simulink model "simulink_pa_lqr_based"  (R2016b)
settings: Solver=FixedStepAuto  StartTime=0.0  StopTime=1  FixedStep=Splant  RelTol=1e-3
undefined symbols (not defined in the file): Ad_plant, application_delay, Bd_plant, Cd_plant, Dd_plant, FForward, Ks, reference, sp_indexes_LPTV, SP_LPTV, sp_samples_in_Sp, Splant
settings Model: SimulationMode=accelerator  SnapshotInterval=2  Creator=juan  LastModifiedBy=jvalencia

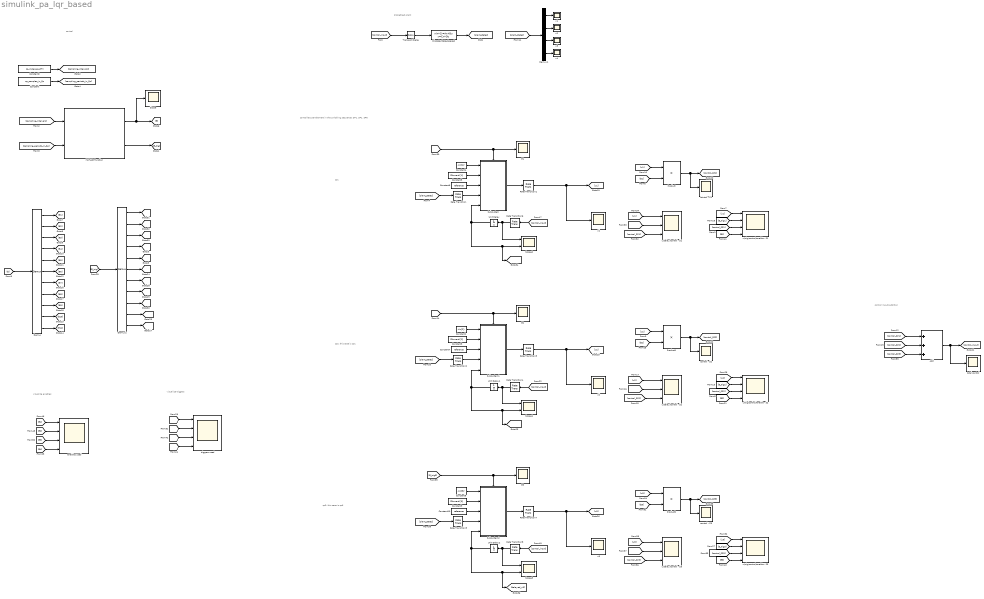
== system simulink_pa_lqr_based ==
  note: discretized plant
  note: control
  note: sp1
  note: control inputs addition
  note: sp2: this case is sp1
  note: sp3: this case is sp6
  note: visualize enables
  note: visualize triggers
  note: controllers per element in the switching sequence:
      | SP1, SP1, SP6
  Add : Sum  Inputs=+++
  Constant : Constant  Value=sp_samples_in_Sp  SampleTime=Splant
  Constant1 : Constant  Value=-Ks{2}  SampleTime=-1
  Constant10 : Constant  Value=reference  SampleTime=-1
  Constant2 : Constant  Value=sp_indexes_LPTV  SampleTime=Splant
  Constant3 : Constant  Value=FForward{2}  SampleTime=-1
  Constant4 : Constant  Value=-Ks{1}  SampleTime=-1
  Constant5 : Constant  Value=FForward{1}  SampleTime=-1
  Constant6 : Constant  Value=reference  SampleTime=-1
  Constant7 : Constant  Value=reference  SampleTime=-1
  Constant8 : Constant  Value=-Ks{3}  SampleTime=-1
  Constant9 : Constant  Value=FForward{3}  SampleTime=-1
  Demux : Demux  Outputs=11
  Demux1 : Demux
  Demux2 : Demux  Outputs=11
  Discrete State-Space2 : DiscreteStateSpace  A=Ad_plant  B=Bd_plant  C=Cd_plant  D=Dd_plant  SampleTime=Splant
  E1 : Scope
  E2 : Scope
  E3 : Scope
  MATLAB Function : MATLAB Function  TreatAsAtomicUnit=on  SystemSampleTime=Splant
  Product : Product
  Product1 : Product
  Product2 : Product
  Rate Transition{,1..4,6} (6 alike) : RateTransition  OutPortSampleTime=SP_LPTV(1)
  Rate Transition5 : RateTransition  OutPortSampleTime=SP_LPTV(2)
  Rate Transition7 : RateTransition  OutPortSampleTime=SP_LPTV(2)
  Rate Transition8 : RateTransition  OutPortSampleTime=SP_LPTV(2)
  Scope : Scope
  Scope1 : Scope  NumInputPorts=2
  Scope2 : Scope  NumInputPorts=2
  Scope3 : Scope  NumInputPorts=2
  Subsystem : Subsystem
  Subsystem1 : Subsystem
  Subsystem2 : Subsystem
  Transport Delay : TransportDelay  DelayTime=application_delay
  Unit Delay : UnitDelay  SampleTime=SP_LPTV(1)
  Unit Delay1 : UnitDelay  SampleTime=SP_LPTV(1)
  Unit Delay2 : UnitDelay  SampleTime=SP_LPTV(2)
  control - S1 : Scope
  control - S2 : Scope
  control - S3 : Scope
  enables used : Scope  NumInputPorts=4
  total control : Scope
  triggers used : Scope  NumInputPorts=4
  u/delay/control - S1 : Scope  NumInputPorts=3
  u/delay/control - S2 : Scope  NumInputPorts=3
  u/delay/control - S3 : Scope  NumInputPorts=3
  u/trig/control/enable - S1 : Scope  NumInputPorts=4
  u/trig/control/enable - S2 : Scope  NumInputPorts=4
  u/trig/control/enable - S3 : Scope  NumInputPorts=4
  u1 : Scope
  u2 : Scope
  u3 : Scope
  x{1..4} (4 alike) : Scope
  wires:
  Discrete State-Space2/1 -> [plant_states]
  [control_input] -> Transport Delay/1
  Constant/1 -> [sampling_periods_in_Sp]
  Constant2/1 -> [sampling_intervals]
  [sampling_periods_in_Sp] -> MATLAB Function/2(sampling_periods_in_Sp)
  [sampling_intervals] -> MATLAB Function/1(sampling_intervals)
  MATLAB Function/1(E_out) -> Scope/1, [E]
  Demux/1 -> [E1]  "E1"
  Demux/2 -> [E2]  "E2"
  Demux/3 -> [E3]  "E3"
  Demux/4 -> [E4]  "E4"
  Demux/5 -> [E5]  "E5"
  Demux/6 -> [E6]  "E6"
  Demux/7 -> [E7]  "E7"
  Demux/8 -> [E8]  "E8"
  Demux/9 -> [E9]  "E9"
  Demux/10 -> [E10]  "E10"
  Demux/11 -> [E11]  "E11"
  Constant4/1 -> Subsystem/1(In1)
  Constant5/1 -> Subsystem/2(In2)
  Constant6/1 -> Subsystem/3(In3)
  [plant_states] -> Rate Transition/1
  [plant_states] -> Demux1/1
  Demux1/1 -> x1/1
  Demux1/2 -> x2/1
  Demux1/3 -> x3/1
  Demux1/4 -> x4/1
  Add/1 -> total control/1, [control_input]
  [control_SP1] -> Add/1
  [u1] -> Product/1
  [E1] -> Product/2
  Product/1 -> control - S1/1, [control_SP1]
  Rate Transition/1 -> Subsystem/4(In4)
  [u1] -> u/trig/control/enable - S1/1
  [E_trig1] -> u/trig/control/enable - S1/2
  [control_SP1] -> u/trig/control/enable - S1/3
  MATLAB Function/2(E_trig_out) -> [E_trig]
  Demux2/1 -> [E_trig1]  "T1"
  Demux2/2 -> [E_trig2]  "T2"
  Demux2/3 -> [E_trig3]  "T3"
  Demux2/4 -> [E_trig4]  "T4"
  Demux2/5 -> [E_trig5]  "T5"
  Demux2/6 -> [E_trig6]  "T6"
  Demux2/7 -> [E_trig7]  "T7"
  Demux2/8 -> [E_trig8]  "T8"
  Demux2/9 -> [E_trig9]  "T9"
  Demux2/10 -> [E_trig10]  "T10"
  Demux2/11 -> [E_trig11]  "T11"
  Unit Delay/1 -> [delayed_u1], Scope2/2, Subsystem/5(In5)
  [E1] -> u/trig/control/enable - S1/4
  Subsystem/1(Out1) -> Rate Transition1/1
  [E_trig1] -> Subsystem/Trigger, E1/1
  [E1] -> enables used/1
  [E2] -> enables used/2
  [E3] -> enables used/3
  [control_input] -> Rate Transition6/1
  Rate Transition6/1 -> Scope2/1, Unit Delay/1
  Rate Transition1/1 -> [u1], u1/1
  Constant1/1 -> Subsystem1/1(In1)
  Constant3/1 -> Subsystem1/2(In2)
  Constant7/1 -> Subsystem1/3(In3)
  [plant_states] -> Rate Transition2/1
  [u2] -> Product1/1
  [E2] -> Product1/2
  Product1/1 -> control - S2/1, [control_SP2]
  Rate Transition2/1 -> Subsystem1/4(In4)
  [u2] -> u/trig/control/enable - S2/1
  [E_trig2] -> u/trig/control/enable - S2/2
  [control_SP2] -> u/trig/control/enable - S2/3
  Unit Delay1/1 -> [delayed_u2], Scope1/2, Subsystem1/5(In5)
  [E2] -> u/trig/control/enable - S2/4
  Subsystem1/1(Out1) -> Rate Transition3/1
  [E_trig2] -> Subsystem1/Trigger, E2/1
  [control_input] -> Rate Transition4/1
  Rate Transition4/1 -> Scope1/1, Unit Delay1/1
  Rate Transition3/1 -> [u2], u2/1
  Transport Delay/1 -> Discrete State-Space2/1
  [control_SP2] -> Add/2
  Constant8/1 -> Subsystem2/1(In1)
  Constant9/1 -> Subsystem2/2(In2)
  Constant10/1 -> Subsystem2/3(In3)
  [plant_states] -> Rate Transition5/1
  [u3] -> Product2/1
  [E3] -> Product2/2
  Product2/1 -> control - S3/1, [control_SP3]
  Rate Transition5/1 -> Subsystem2/4(In4)
  [u3] -> u/trig/control/enable - S3/1
  [E_trig3] -> u/trig/control/enable - S3/2
  [control_SP3] -> u/trig/control/enable - S3/3
  Unit Delay2/1 -> [delayed_u3], Scope3/2, Subsystem2/5(In5)
  [u3] -> u/delay/control - S3/1
  [delayed_u3] -> u/delay/control - S3/2
  [control_SP3] -> u/delay/control - S3/3
  [E3] -> u/trig/control/enable - S3/4
  Subsystem2/1(Out1) -> Rate Transition7/1
  [E_trig3] -> Subsystem2/Trigger, E3/1
  [control_input] -> Rate Transition8/1
  Rate Transition8/1 -> Scope3/1, Unit Delay2/1
  Rate Transition7/1 -> [u3], u3/1
  [control_SP3] -> Add/3
  [E] -> Demux/1
  [E_trig] -> Demux2/1
  [E4] -> enables used/4
  [E_trig1] -> triggers used/1
  [E_trig2] -> triggers used/2
  [E_trig3] -> triggers used/3
  [E_trig4] -> triggers used/4
  [u2] -> u/delay/control - S2/1
  [delayed_u2] -> u/delay/control - S2/2
  [control_SP2] -> u/delay/control - S2/3
  [u1] -> u/delay/control - S1/1
  [delayed_u1] -> u/delay/control - S1/2
  [control_SP1] -> u/delay/control - S1/3

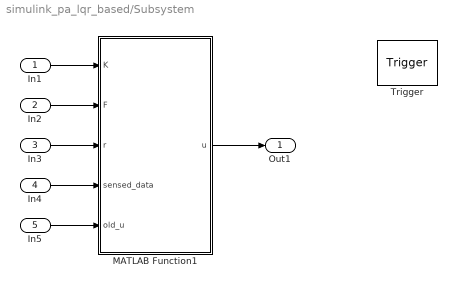
== system simulink_pa_lqr_based/Subsystem ==
  In1 : Inport
  In2 : Inport  Port=2
  In3 : Inport  Port=3
  In4 : Inport  Port=4
  In5 : Inport  Port=5
  Trigger : TriggerPort  VariantControl=Variant  PortDimensions=1
  MATLAB Function1 : MATLAB Function  TreatAsAtomicUnit=on
  Out1 : Outport
  wires:
  In1/1 -> MATLAB Function1/1(K)
  In3/1 -> MATLAB Function1/3(r)
  In2/1 -> MATLAB Function1/2(F)
  In4/1 -> MATLAB Function1/4(sensed_data)
  MATLAB Function1/1(u) -> Out1/1
  In5/1 -> MATLAB Function1/5(old_u)

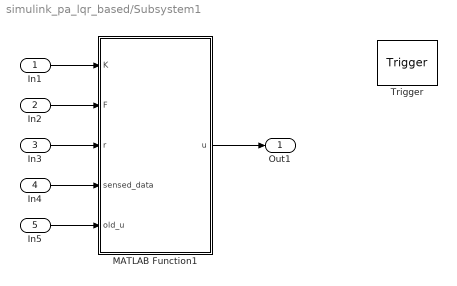
== system simulink_pa_lqr_based/Subsystem1 ==
  In1 : Inport
  In2 : Inport  Port=2
  In3 : Inport  Port=3
  In4 : Inport  Port=4
  In5 : Inport  Port=5
  Trigger : TriggerPort  VariantControl=Variant  PortDimensions=1
  MATLAB Function1 : MATLAB Function  TreatAsAtomicUnit=on
  Out1 : Outport
  wires:
  In1/1 -> MATLAB Function1/1(K)
  In3/1 -> MATLAB Function1/3(r)
  In2/1 -> MATLAB Function1/2(F)
  In4/1 -> MATLAB Function1/4(sensed_data)
  MATLAB Function1/1(u) -> Out1/1
  In5/1 -> MATLAB Function1/5(old_u)

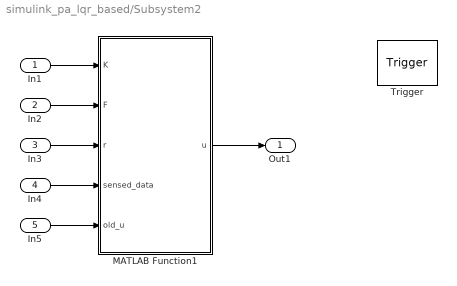
== system simulink_pa_lqr_based/Subsystem2 ==
  In1 : Inport
  In2 : Inport  Port=2
  In3 : Inport  Port=3
  In4 : Inport  Port=4
  In5 : Inport  Port=5
  Trigger : TriggerPort  VariantControl=Variant  PortDimensions=1
  MATLAB Function1 : MATLAB Function  TreatAsAtomicUnit=on
  Out1 : Outport
  wires:
  In1/1 -> MATLAB Function1/1(K)
  In3/1 -> MATLAB Function1/3(r)
  In2/1 -> MATLAB Function1/2(F)
  In4/1 -> MATLAB Function1/4(sensed_data)
  MATLAB Function1/1(u) -> Out1/1
  In5/1 -> MATLAB Function1/5(old_u)

== matlab function simulink_pa_lqr_based/Subsystem/MATLAB Function1 ==
  data: K input; F input; r input; u output; sensed_data input; old_u input
function u = control(K, F, r, sensed_data, old_u)

z = [sensed_data; old_u];
u = K'*z + F*r;

== matlab function simulink_pa_lqr_based/MATLAB Function ==
  data: sampling_intervals input; sampling_periods_in_Sp input; E_out output; E_trig_out output
function [E_out,E_trig_out]  = switching_control_calculation(sampling_intervals, sampling_periods_in_Sp)

% slots
N = 10;
max_sampling_periods = N+1;

% index
persistent index;
if (isempty(index)) %It does not already exist
    index = 1; % initialize with index 1
end

% index_old
persistent index_old;
if (isempty(index_old)) %It does not already exist
    index_old = 1; % initialize with index 1
end

% loop
persistent loop;
if (isempty(loop)) %It does not already exist
    loop = 1; % initialize with loop 1 
end
    
% E
persistent E;
if (isempty(E))
    E = zeros(1, max_sampling_periods);
end

% E_trig
persistent E_trig;
if (isempty(E_trig))
    E_trig = zeros(1, max_sampling_periods);
end

% E_old
persistent E_old;
if (isempty(E_old))
    E_old = zeros(1, max_sampling_periods);
end


% initialization variable: test
persistent test;
if (isempty(test)) %It does not already exist
    test = 1; % initialize with loop 1 
    E_out       = zeros(1, max_sampling_periods); % enable
    E_trig_out  = zeros(1, max_sampling_periods); % trigger
else
    
    if loop < sampling_periods_in_Sp(index)
        loop = loop + 1;
    else
        loop = 1;

        if index < length(sampling_periods_in_Sp)
            index = index + 1;
        else
            index = 1;
        end
    end
    
    % SP1, SP2, SP10
    for i = 1:max_sampling_periods
        if(sampling_intervals(index) == i)
            % setting regular enable
            E(i) = 1;
            
            % setting triggereing enable
            if (index ~= index_old)
                if (E_old(i) == 1)
                    E_trig(i) = 0;
                else
                    E_trig(i) = 1;
                end       
            else
                E_trig(i) = 0;
                
                if (loop == 2) % just for the first mode
                    E_trig(i) = 1;
                else
                    E_trig(i) = 0;
                end
            end
            
        else
            E(i) = 0;
            E_trig(i) = 0;
        end
        
        E_old(i) = E_trig(i);
    end

    index_old  = index;
    
    % setting values of enable and trigger
    E_out      = E;
    E_trig_out = E_trig;
   
end

== matlab function simulink_pa_lqr_based/Subsystem1/MATLAB Function1 ==
  data: K input; F input; r input; u output; sensed_data input; old_u input
function u = control(K, F, r, sensed_data, old_u)

z = [sensed_data; old_u];
u = K'*z + F*r;

== matlab function simulink_pa_lqr_based/Subsystem2/MATLAB Function1 ==
  data: K input; F input; r input; u output; sensed_data input; old_u input
function u = control(K, F, r, sensed_data, old_u)

z = [sensed_data; old_u];
u = K'*z + F*r;
